simulink model "fitts_bimanual"  (Simulink 7.0)
settings: Solver=ode4  SolverMode=SingleTasking  StartTime=0.0  StopTime=inf  FixedStep=0.0005  RelTol=1e-3
undefined symbols (not defined in the file or in its folder): slselsubs
libraries: dspbuff3 x2, General x2, Video x1
settings Model: Creator=Administrator  LastModifiedBy=Administrator  BufferReuse=off
settings OptimizationCC: BlockReduction=off  OptimizeBlockIOStorage=off  BufferReuse=off  ExpressionFolding=off  LocalBlockOutputs=off
settings HardwareCC: ProdIntDivRoundTo=Floor  ProdEndianess=LittleEndian  ProdHWDeviceType=Intel->x86/Pentium  TargetHWDeviceType=32-bit Generic  ProdEqTarget=off
settings RTWCC: SystemTargetFile=xpctarget.tlc  TemplateMakefile=xpc_default_tmf  Description=xPC Target  ProcessScript=xpctarget_make_rtw_hook
settings xpcTargetCC: TargetFcnLib=ansi_tfl_table_tmw.mat  GenFloatMathFcnCalls=ANSI_C  CompOptLevelCompliant=off  PortableWordSizes=off  xPCisDownloadable=off

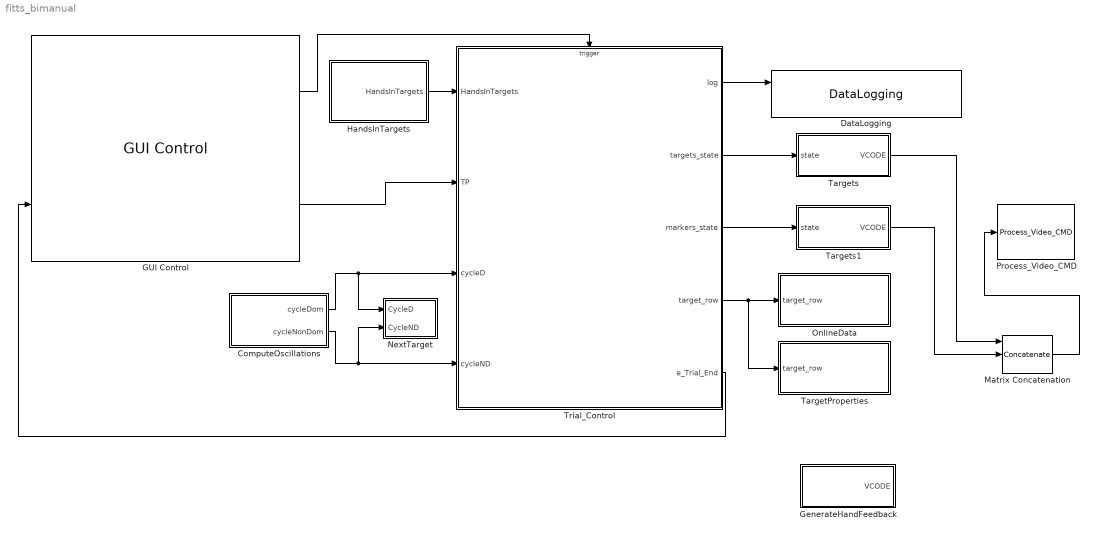
== system fitts_bimanual ==
  ComputeOscillations : Subsystem
  DataLogging : General/DataLogging  SystemSampleTime=-1  log_event_codes=on  log_analog_inputs=off
  GUI Control : General/GUI Control  SystemSampleTime=-1  target_type_str=Circle  Target_Type=1  XYcols=[1 2]  Vcols=3  Lcols=4  indices_padding=[0 0 0 0;0 0 0 0]  show_repeat_trial_flag=on
  GenerateHandFeedback : Subsystem
  HandsInTargets : Subsystem
  Matrix Concatenation : Concatenate  NumInputs=3  Mode=Multidimensional array
  NextTarget : Subsystem
  OnlineData : Subsystem
  Process_Video_CMD : Video/Process_Video_CMD  SystemSampleTime=-1
  TargetProperties : Subsystem
  Targets : Subsystem
  Targets1 : Subsystem
  Trial_Control : Stateflow chart
  wires:
  Matrix Concatenation/1 -> Process_Video_CMD/1
  Targets/1(VCODE) -> Matrix Concatenation/1
  GUI Control/1 -> Trial_Control/Trigger
  Trial_Control/5(e_Trial_End) -> GUI Control/2
  HandsInTargets/1(HandsInTargets) -> Trial_Control/1(HandsInTargets)
  GUI Control/2 -> Trial_Control/2(TP)
  Targets1/1(VCODE) -> Matrix Concatenation/2
  Trial_Control/2(targets_state) -> Targets/1(state)
  Trial_Control/3(markers_state) -> Targets1/1(state)
  Trial_Control/1(log) -> DataLogging/1
  ComputeOscillations/2(cycleNonDom) -> Trial_Control/4(cycleND), NextTarget/2(CycleND)
  ComputeOscillations/1(cycleDom) -> Trial_Control/3(cycleD), NextTarget/1(CycleD)
  Trial_Control/4(target_row) -> TargetProperties/1(target_row), OnlineData/1(target_row)

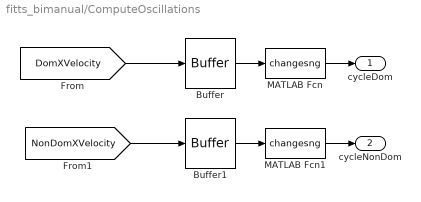
== system fitts_bimanual/ComputeOscillations ==
  Buffer : dspbuff3/Buffer  N=10  V=10  ic=0
  Buffer1 : dspbuff3/Buffer  N=10  V=10  ic=0
  MATLAB Fcn : MATLABFcn  MATLABFcn=changesng
  MATLAB Fcn1 : MATLABFcn  MATLABFcn=changesng
  cycleDom : Outport  OutDataType=sfix(16)  OutScaling=2^0
  cycleNonDom : Outport  Port=2  OutDataType=sfix(16)  OutScaling=2^0
  wires:
  Buffer/1 -> MATLAB Fcn/1
  MATLAB Fcn/1 -> cycleDom/1
  Buffer1/1 -> MATLAB Fcn1/1
  MATLAB Fcn1/1 -> cycleNonDom/1
  [DomXVelocity] -> Buffer/1
  [NonDomXVelocity] -> Buffer1/1

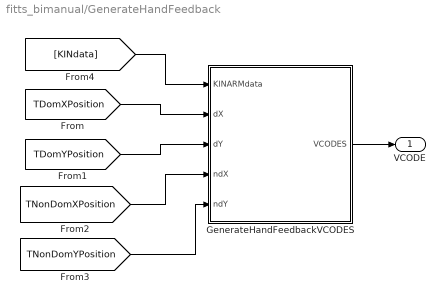
== system fitts_bimanual/GenerateHandFeedback ==
  GenerateHandFeedbackVCODES : Stateflow chart
  VCODE : Outport
  wires:
  GenerateHandFeedbackVCODES/1(VCODES) -> VCODE/1
  [KINdata] -> GenerateHandFeedbackVCODES/1(KINARMdata)
  [TDomXPosition] -> GenerateHandFeedbackVCODES/2(dX)
  [TDomYPosition] -> GenerateHandFeedbackVCODES/3(dY)
  [TNonDomXPosition] -> GenerateHandFeedbackVCODES/4(ndX)
  [TNonDomYPosition] -> GenerateHandFeedbackVCODES/5(ndY)

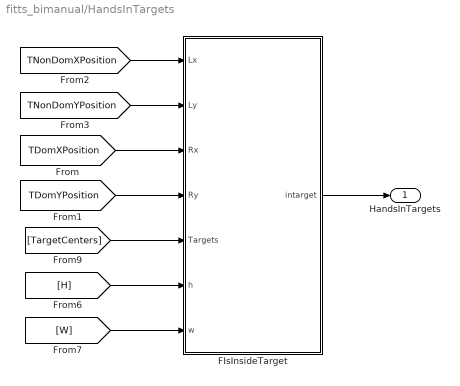
== system fitts_bimanual/HandsInTargets ==
  FIsInsideTarget : Stateflow chart
  HandsInTargets : Outport
  wires:
  [TargetCenters] -> FIsInsideTarget/5(Targets)
  [H] -> FIsInsideTarget/6(h)
  [W] -> FIsInsideTarget/7(w)
  FIsInsideTarget/1(intarget) -> HandsInTargets/1
  [TNonDomXPosition] -> FIsInsideTarget/1(Lx)
  [TNonDomYPosition] -> FIsInsideTarget/2(Ly)
  [TDomXPosition] -> FIsInsideTarget/3(Rx)
  [TDomYPosition] -> FIsInsideTarget/4(Ry)

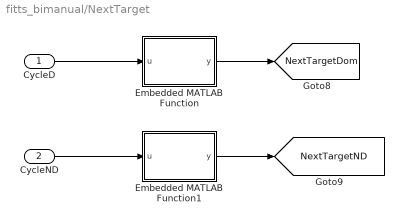
== system fitts_bimanual/NextTarget ==
  CycleD : Inport
  CycleND : Inport  Port=2
  Embedded MATLAB Function : Stateflow chart
  Embedded MATLAB Function1 : Stateflow chart
  tag scope: NextTargetDom=global, NextTargetND=global
  wires:
  CycleD/1 -> Embedded MATLAB Function/1(u)
  CycleND/1 -> Embedded MATLAB Function1/1(u)
  Embedded MATLAB Function/1(y) -> [NextTargetDom]
  Embedded MATLAB Function1/1(y) -> [NextTargetND]

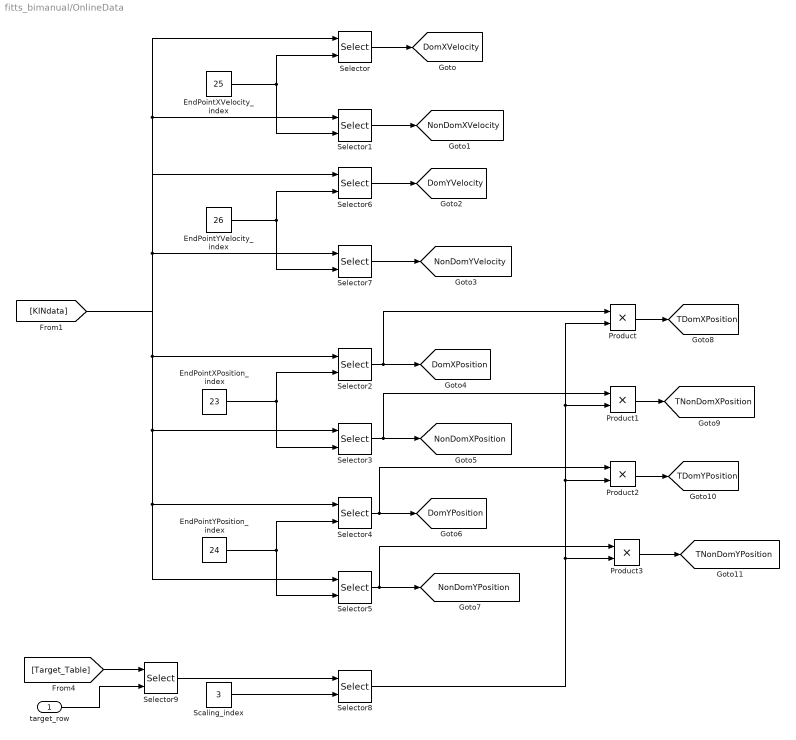
== system fitts_bimanual/OnlineData ==
  target_row : Inport  OutDataType=sfix(16)  OutScaling=2^0
  EndPointXPosition_index : Constant  Value=23  OutDataType=sfix(16)  OutScaling=2^0
  EndPointXVelocity_index : Constant  Value=25  OutDataType=sfix(16)  OutScaling=2^0
  EndPointYPosition_index : Constant  Value=24  OutDataType=sfix(16)  OutScaling=2^0
  EndPointYVelocity_index : Constant  Value=26  OutDataType=sfix(16)  OutScaling=2^0
  Product{,1..3} (4 alike) : Product  OutDataType=sfix(16)  OutScaling=2^0  RndMeth=Zero
  Scaling_index : Constant  Value=3  OutDataType=sfix(16)  OutScaling=2^0
  Selector{,2,4,6,8..9} (6 alike) : Selector  NumberOfDimensions=2  InputPortWidth=3  IndexOptions=Index vector (port),Index vector (dialog)  Indices=1,1  OutputSizes=slselsubs([(-2),(-2)],1),slselsubs([(-2),(-2)],2)
  Selector{1,3,5,7} (4 alike) : Selector  NumberOfDimensions=2  InputPortWidth=3  IndexOptions=Index vector (port),Index vector (dialog)  Indices=1,2  OutputSizes=slselsubs([(-2),(-2)],1),slselsubs([(-2),(-2)],2)
  tag scope: DomXPosition=global, DomXVelocity=global, DomYPosition=global, DomYVelocity=global, NonDomXPosition=global, NonDomXVelocity=global, NonDomYPosition=global, NonDomYVelocity=global, TDomXPosition=global, TDomYPosition=global, TNonDomXPosition=global, TNonDomYPosition=global
  wires:
  [KINdata] -> Selector1/1, Selector/1, Selector2/1, Selector3/1, Selector4/1, Selector5/1, Selector6/1, Selector7/1
  Selector3/1 -> [NonDomXPosition], Product1/1
  Selector/1 -> [DomXVelocity]
  EndPointXVelocity_index/1 -> Selector/2, Selector1/2
  Selector1/1 -> [NonDomXVelocity]
  EndPointXPosition_index/1 -> Selector2/2, Selector3/2
  Selector2/1 -> [DomXPosition], Product/1
  Selector5/1 -> [NonDomYPosition], Product3/1
  EndPointYPosition_index/1 -> Selector4/2, Selector5/2
  Selector4/1 -> [DomYPosition], Product2/1
  Selector6/1 -> [DomYVelocity]
  EndPointYVelocity_index/1 -> Selector6/2, Selector7/2
  Selector7/1 -> [NonDomYVelocity]
  Product/1 -> [TDomXPosition]
  Product1/1 -> [TNonDomXPosition]
  Product2/1 -> [TDomYPosition]
  Product3/1 -> [TNonDomYPosition]
  Scaling_index/1 -> Selector8/2
  Selector8/1 -> Product/2, Product1/2, Product2/2, Product3/2
  Selector9/1 -> Selector8/1
  [Target_Table] -> Selector9/1
  target_row/1 -> Selector9/2

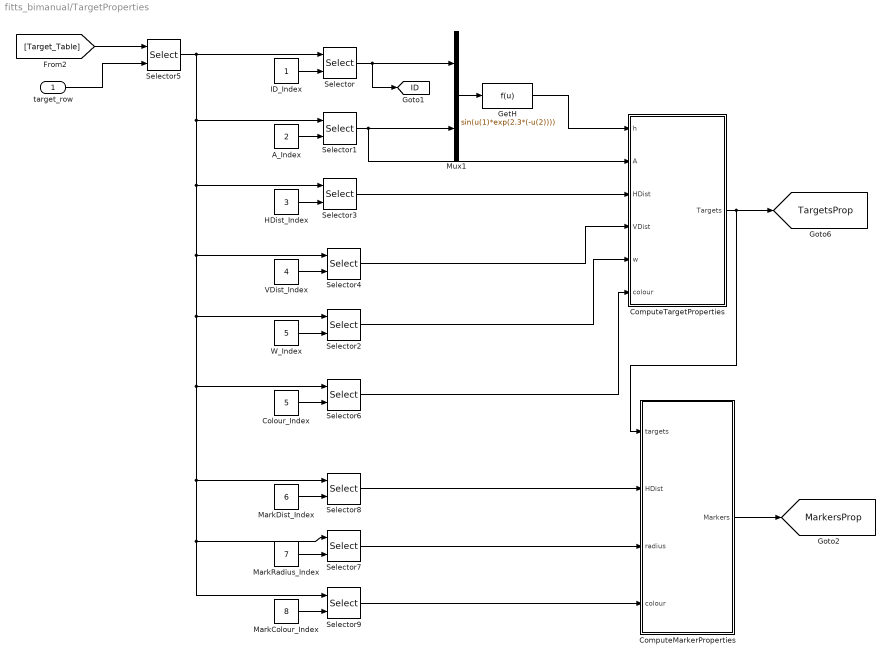
== system fitts_bimanual/TargetProperties ==
  target_row : Inport  OutDataType=sfix(16)  OutScaling=2^0
  A_Index : Constant  Value=2  OutDataType=sfix(16)  OutScaling=2^0
  Colour_Index : Constant  Value=5  OutDataType=sfix(16)  OutScaling=2^0
  ComputeMarkerProperties : Stateflow chart
  ComputeTargetProperties : Stateflow chart
  GetH : Fcn  Expr=sin(u(1)*exp(2.3*(-u(2))))
  HDist_Index : Constant  Value=3  OutDataType=sfix(16)  OutScaling=2^0
  ID_Index : Constant  OutDataType=sfix(16)  OutScaling=2^0
  MarkColour_Index : Constant  Value=8  OutDataType=sfix(16)  OutScaling=2^0
  MarkDist_Index : Constant  Value=6  OutDataType=sfix(16)  OutScaling=2^0
  MarkRadius_Index : Constant  Value=7  OutDataType=sfix(16)  OutScaling=2^0
  Mux1 : Mux  Inputs=2
  Selector{,1..9} (10 alike) : Selector  NumberOfDimensions=2  InputPortWidth=3  IndexOptions=Index vector (port),Index vector (dialog)  Indices=1,1  OutputSizes=slselsubs([(-2),(-2)],1),slselsubs([(-2),(-2)],2)
  VDist_Index : Constant  Value=4  OutDataType=sfix(16)  OutScaling=2^0
  W_Index : Constant  Value=5  OutDataType=sfix(16)  OutScaling=2^0
  tag scope: ID=global, MarkersProp=global, TargetsProp=global
  wires:
  ID_Index/1 -> Selector/2
  Selector5/1 -> Selector/1, Selector1/1, Selector3/1, Selector4/1, Selector2/1, Selector6/1, Selector8/1, Selector7/1, Selector9/1
  A_Index/1 -> Selector1/2
  HDist_Index/1 -> Selector3/2
  VDist_Index/1 -> Selector4/2
  Mux1/1 -> GetH/1
  Selector/1 -> Mux1/1, [ID]
  Selector1/1 -> Mux1/2, ComputeTargetProperties/2(A)
  Selector3/1 -> ComputeTargetProperties/3(HDist)
  Selector4/1 -> ComputeTargetProperties/4(VDist)
  ComputeTargetProperties/1(Targets) -> [TargetsProp], ComputeMarkerProperties/1(targets)
  W_Index/1 -> Selector2/2
  Selector2/1 -> ComputeTargetProperties/5(w)
  Colour_Index/1 -> Selector6/2
  Selector6/1 -> ComputeTargetProperties/6(colour)
  GetH/1 -> ComputeTargetProperties/1(h)
  [Target_Table] -> Selector5/1
  target_row/1 -> Selector5/2
  MarkDist_Index/1 -> Selector8/2
  MarkRadius_Index/1 -> Selector7/2
  MarkColour_Index/1 -> Selector9/2
  Selector8/1 -> ComputeMarkerProperties/2(HDist)
  Selector7/1 -> ComputeMarkerProperties/3(radius)
  Selector9/1 -> ComputeMarkerProperties/4(colour)
  ComputeMarkerProperties/1(Markers) -> [MarkersProp]

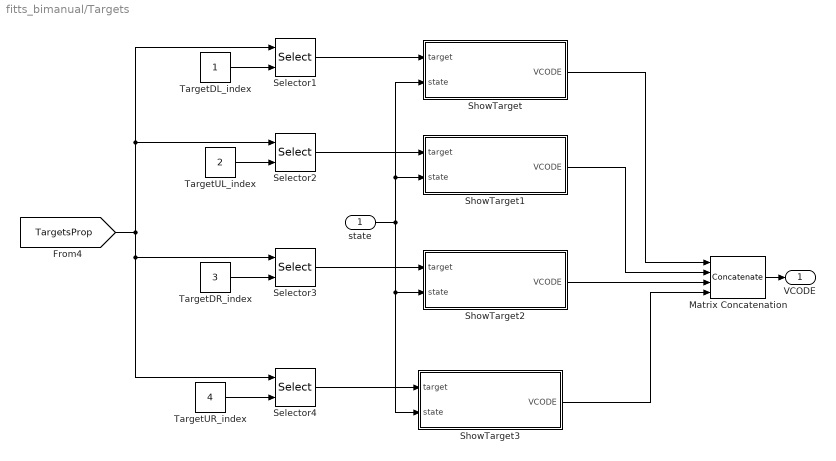
== system fitts_bimanual/Targets ==
  state : Inport
  Matrix Concatenation : Concatenate  NumInputs=4  Mode=Multidimensional array
  Selector{1..4} (4 alike) : Selector  NumberOfDimensions=2  InputPortWidth=3  IndexOptions=Index vector (port),Index vector (dialog)  Indices=1,2  OutputSizes=slselsubs([(-2),(-2)],1),slselsubs([(-2),(-2)],2)
  ShowTarget : Stateflow chart
  ShowTarget1 : Stateflow chart
  ShowTarget2 : Stateflow chart
  ShowTarget3 : Stateflow chart
  TargetDL_index : Constant  OutDataType=sfix(16)  OutScaling=2^0
  TargetDR_index : Constant  Value=3  OutDataType=sfix(16)  OutScaling=2^0
  TargetUL_index : Constant  Value=2  OutDataType=sfix(16)  OutScaling=2^0
  TargetUR_index : Constant  Value=4  OutDataType=sfix(16)  OutScaling=2^0
  VCODE : Outport  OutDataType=sfix(16)  OutScaling=2^0
  wires:
  state/1 -> ShowTarget/2(state), ShowTarget1/2(state), ShowTarget2/2(state), ShowTarget3/2(state)
  ShowTarget/1(VCODE) -> Matrix Concatenation/1
  ShowTarget1/1(VCODE) -> Matrix Concatenation/2
  ShowTarget2/1(VCODE) -> Matrix Concatenation/3
  Matrix Concatenation/1 -> VCODE/1
  ShowTarget3/1(VCODE) -> Matrix Concatenation/4
  TargetDL_index/1 -> Selector1/2
  [TargetsProp] -> Selector1/1, Selector2/1, Selector3/1, Selector4/1
  TargetUL_index/1 -> Selector2/2
  TargetDR_index/1 -> Selector3/2
  TargetUR_index/1 -> Selector4/2
  Selector1/1 -> ShowTarget/1(target)
  Selector2/1 -> ShowTarget1/1(target)
  Selector3/1 -> ShowTarget2/1(target)
  Selector4/1 -> ShowTarget3/1(target)

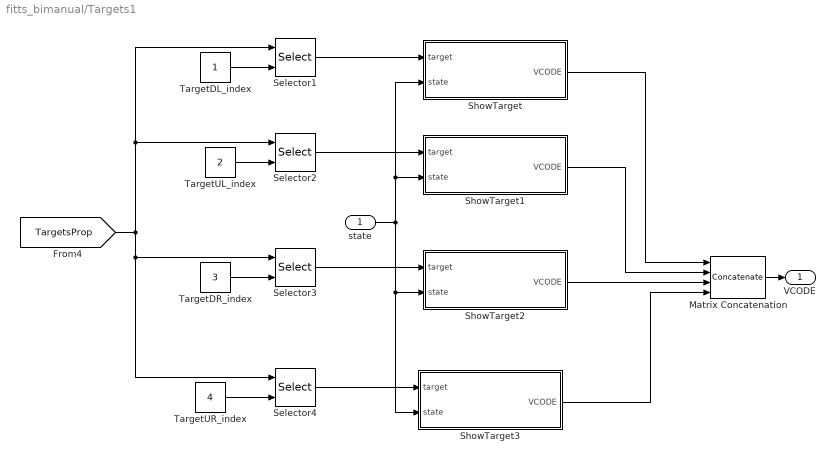
== system fitts_bimanual/Targets1 ==
  state : Inport
  Matrix Concatenation : Concatenate  NumInputs=4  Mode=Multidimensional array
  Selector{1..4} (4 alike) : Selector  NumberOfDimensions=2  InputPortWidth=3  IndexOptions=Index vector (port),Index vector (dialog)  Indices=1,2  OutputSizes=slselsubs([(-2),(-2)],1),slselsubs([(-2),(-2)],2)
  ShowTarget : Stateflow chart
  ShowTarget1 : Stateflow chart
  ShowTarget2 : Stateflow chart
  ShowTarget3 : Stateflow chart
  TargetDL_index : Constant  OutDataType=sfix(16)  OutScaling=2^0
  TargetDR_index : Constant  Value=3  OutDataType=sfix(16)  OutScaling=2^0
  TargetUL_index : Constant  Value=2  OutDataType=sfix(16)  OutScaling=2^0
  TargetUR_index : Constant  Value=4  OutDataType=sfix(16)  OutScaling=2^0
  VCODE : Outport  OutDataType=sfix(16)  OutScaling=2^0
  wires:
  state/1 -> ShowTarget/2(state), ShowTarget1/2(state), ShowTarget2/2(state), ShowTarget3/2(state)
  ShowTarget/1(VCODE) -> Matrix Concatenation/1
  ShowTarget1/1(VCODE) -> Matrix Concatenation/2
  ShowTarget2/1(VCODE) -> Matrix Concatenation/3
  Matrix Concatenation/1 -> VCODE/1
  ShowTarget3/1(VCODE) -> Matrix Concatenation/4
  TargetDL_index/1 -> Selector1/2
  [TargetsProp] -> Selector1/1, Selector2/1, Selector3/1, Selector4/1
  TargetUL_index/1 -> Selector2/2
  TargetDR_index/1 -> Selector3/2
  TargetUR_index/1 -> Selector4/2
  Selector1/1 -> ShowTarget/1(target)
  Selector2/1 -> ShowTarget1/1(target)
  Selector3/1 -> ShowTarget2/1(target)
  Selector4/1 -> ShowTarget3/1(target)

== stateflow chart Trial_Control ==
  state Initialize/
    log=0
  state Wait4Subject/
    //Turn on markers and targets with specified size
    targets_state=1
    markers_state=1
    log=0
    oscillations=0
  state PreOscillationDelay/
    //Wait specified period of time
    delay=TP[0]
  state Oscillate/
    //Hold oscillation until subject reaches trial limit
    markers_state=0
    log=1
  state EndOfTrial/
    //Wait specified period of time
    delay=TP[0]
    targets_state=0
  state InterTrial/
    //Set up new
    e_Trial_End
    delay=TP[0]
  Wait4Subject -> PreOscillationDelay : [HandsInTargets]
  PreOscillationDelay -> Oscillate : after(delay,e_clk)
  Initialize -> Wait4Subject
  Oscillate -> EndOfTrial : [oscillations=TP[0]]
  EndOfTrial -> InterTrial
  InterTrial -> Wait4Subject : after(delay,e_clk)
  (default) -> Initialize : //init task
  data: log output boolean; HandsInTargets input inherited; TP input inherited; cycleD input inherited; targets_state output boolean; markers_state output double; cycleND input inherited; PREOSCDELAY_COL constant uint8 =1; INTERTRIALDELAY_COL constant uint8 =2; FEEDBACKSCALING_COL constant uint8 =3; target_row output double
  events: e_clk input RISING_EDGE_EVENT; e_ExitTrialNow input EITHER_EDGE_EVENT; e_Trial_End output EITHER_EDGE_EVENT

== matlab function NextTarget/Embedded MATLAB Function ==
  data: u input inherited; y output inherited
function y = fcn(u)
% This block supports the Embedded MATLAB subset.
% See the help menu for details. 

y = u;

== matlab function NextTarget/Embedded MATLAB Function1 ==
  data: u input inherited; y output inherited
function y = fcn(u)
% This block supports the Embedded MATLAB subset.
% See the help menu for details. 

y = u;

== matlab function GenerateHandFeedback/GenerateHandFeedbackVCODES ==
  data: KINARMdata input inherited; VCODES output inherited; dX input inherited; dY input inherited; ndX input inherited; ndY input inherited
function VCODES  = fcn(KINARMdata,dX,dY,ndX,ndY)
%
% This function creates the VCODEs for the hand position feedback for both
% hands.  Various options in the Mask of the Simulink block in which this
% embedded Matlab file sits, allow the user to specify how often
% the hand feedback is updated as well as the source of the style and status
% of the hand feedback.  


dominant_arm=KINARMdata(3,1);
feedfwd=KINARMdata(3,2);				%amount of feedforward extrapolation for hand position(s)
fdbk_stts_GUI=KINARMdata(3,3);			%status of hand feedback requested from GUI
fdbk_src_GUI=KINARMdata(3,4);			%source of hand feedback style requested from GUI
fdbk_clr_GUI=KINARMdata(3,5);			%colour of hand feedback required by GUI
fdbk_radius_GUI=KINARMdata(3,6);		%radius of hand feedback required by GUI


%----------------Feedback Style ----------------
VCODES=zeros(2,20);						%set default
VCODES(:,1)=1;							%target_type of circle
VCODES(:,5)=fdbk_clr_GUI;				%fill colour as specified by GUI
VCODES(:,6)=fdbk_clr_GUI;				%stroke colour same as fill colour
VCODES(:,7)=0;							%no stroke width
VCODES(:,10)=fdbk_radius_GUI;			%radius (m) as specified by GUI

%show both hand feedbacks
VCODES(1,2)=1;
VCODES(2,2)=1;
end

%----------------Feedback Position ----------------
%set the position of the hand feedback.
for i=1:2
	if i==1
		active_arm=KINARMdata(3,1);			%choose dominant arm first
	else
		active_arm=3-KINARMdata(3,1);		%choose non-dominant arm 2nd
	end
	HandXPos=KINARMdata(active_arm,23);		%(m)
	HandYPos=KINARMdata(active_arm,24);		%(m)
	HandXVel=KINARMdata(active_arm,25);		%(m/s)
	HandYVel=KINARMdata(active_arm,26);		%(m/s)

	% feed-forward hand position (m)
	HandXPos_ff = HandXPos + HandXVel*feedfwd;
	HandYPos_ff = HandYPos + HandYVel*feedfwd;
	VCODES(i,3)=HandXPos_ff;				%target position in m 
	VCODES(i,4)=HandYPos_ff;				%target position in m 
end

VCODES_out=VCODES;

== matlab function TargetProperties/ComputeMarkerProperties ==
  data: targets input inherited; HDist input inherited; radius input inherited; Markers output inherited; colour input inherited
function Markers = fcn(targets,HDist,radius,colour)
% This block supports the Embedded MATLAB subset.
% See the help menu for details. 

% Components of the returned arrays: FORGET ABOUT IT!!!
% X0[1,:] -> Dominant arm
% X0[2,:] -> Non Dominant arm
% X0[:,1] -> Lower targets
% X0[:,2] -> Upper targets

% New version:
% Targets:[ x1, y1, w, h, colour]  Left Down
%         [ x2, y2, w, h, colour]  Left Up
%         [ x3, y3, w, h, colour]  Right Down
%         [ x4, y4, w, h, colour]  Right Up

c=1;  % Distances are in centimeters, need to convert to meters. CHECK UNITS!!!!!

Targets = [ -HDist/2*c, VDist*c,     w, h, colour; ...
            -HDist/2*c, VDist*c+A*c, w, h, colour; ...
             HDist/2*c, VDist*c,     w, h, colour; ...
             HDist/2*c, VDist*c+A*c, w, h, colour];

== matlab function HandsInTargets/FIsInsideTarget ==
  data: Lx input inherited; Ly input inherited; Rx input inherited; Ry input inherited; Targets input inherited; h input inherited; intarget output inherited; w input inherited
function intarget = fcn(Lx,Ly,Rx,Ry,Targets,h,w)
% This block supports the Embedded MATLAB subset.
% See the help menu for details. 

 deltaLx = Lx - Targets(:,1)*0.01;
 deltaLy = Ly - Targets(:,2)*0.01;
 deltaRx = Rx - Targets(:,1)*0.01;
 deltaRy = Ry - Targets(:,2)*0.01;
 
 intarget = zeros(length(Targets),2);
 
 intarget(:,1)= abs(deltaLx) <= w/2 & abs(deltaLy) <= h/2;
 intarget(:,2)= abs(deltaRx) <= w/2 & abs(deltaRy) <= h/2;

== matlab function Targets/ShowTarget1 ==
  data: target input inherited; VCODE output inherited; state input inherited
function VCODE  = fcn(target, state)
% This block supports an embeddable subset of the MATLAB language.
% See the help menu for details. 

% VCODEs are length 20.
% All dimensions are units of (m).
% VCODE index definition: 1-5 as the same for all target types
% 1 - Target type
%		1=circle
%		2=ellipse
%       3=rectangle
%		4=line
%       5=triangle
%		6 and higher - not implemented yet
% 2 - status
%		0=off
%		1=on
% 3 - x position (m)
% 4 - y position (m)
% 5 - fill colour
% 6 - stroke colour
% 7 - stroke width
% 8 - reserved
% 9 - reserved
%
% For circles
% 10 - radius (m)
%
% For ellipses
% 10 - major radius (m)
% 11 - minor radius (m)
% 12 - orientation of major axis (rad)
%
% For rectangles
% 10 - length (m)
% 11 - height (m)
% 12 - orientation (rad) (relative to x,y already shown)
%
% For lines
% 10 - end point x-axis coordinate relative to start point (m)
% 11 - end point y-axis coordinate relative to start point (m)
%
% For triangles
% 10 - length (m)
% 11 - height (m)
% 12 - offset of peak from midpoint of length (m)
% 13 - orientation (rad)

VCODE=zeros(1,20);		%default - target is not defined

if (state==0)
	return;							%state==0 means that the target is off
end

VCODE(1)=3; %They are rectangles

VCODE(2)=1;							%default is that target is 'on'
VCODE(3)=target_pos(0)*0.01;		%target position in target table is cm (v1.4)
VCODE(4)=target_pos(1)*0.01;		%target position in target table is cm (v1.4)

% Fill colour currently comes from the GUI in 1.x format: RRRGGGBBB. Convert this to a 32-bit 
% 0xRRGGBBAA value, or use zero for transparency if target table index for the colour is zero.
if stateindices(state,1)==0
	VCODE(5)=0;
else
	VCODE(5)=colourshift(target(5));			%fill colour
end

% Stroke colour currently comes from the GUI in 1.x format: RRRGGGBBB. Convert this to a 32-bit 
% 0xRRGGBBAA value, or use zero for transparency if target table index for the colour is zero.
% if stateindices(state,2)==0
% 	VCODE(6)=0;				%if stroke-colour column==0, then stroke colour=0
% else
% 	VCODE(6)=colourshift(target(stateindices(state,2)));			%stroke colour
% end

%if target table index for stroke width is zero, then the stroke width is undefined
% if stateindices(state,3)==0
% 	VCODE(7)=0;					%if stroke-width column==0, then stroke width=0
% elseif stateindices(state,3)<0
% 	VCODE(7)=0.001;			%if stroke is not defined, then a 1mm default is chosen
% else
% 	VCODE(7)=target(stateindices(state,3))*0.01;	%stroke width in target table is cm 
% end

VCODE(10)=target(3)*0.01;       %length (m) -- length in target table is in cm
VCODE(11)=target(4)*0.01;       %height (m) -- height in target table is in cm
% if stateindices(state,6)==0
%     VCODE(12)=0;				%if orientation column==0, then orientation=0
% else
%     VCODE(12)=mod(target(stateindices(state,6)),360)*pi/180.0;  %orientation (rad) -- orientation in target table is degrees (v1.4)
% end

%colourshift converts an RRRGGGBBB colour into an RRGBBAA, as an uint32 
function RRGGBBAA = colourshift(RRRGGGBBB)
	blue = cast(mod(RRRGGGBBB,1000),'uint32');
	green= cast(mod(RRRGGGBBB-blue,1000000)/1000,'uint32');
	red  = cast((RRRGGGBBB-green*1000-blue)/1000000,'uint32');
    RRGGBBAA =   bitshift(red,24)...		% red component
				+ bitshift(green,16)...		% green component
				+ bitshift(blue,8)...		% blue component
				+ 255;						% alpha component

== matlab function Targets/ShowTarget2 ==
  data: target input inherited; VCODE output inherited; state input inherited
function VCODE  = fcn(target, state)
% This block supports an embeddable subset of the MATLAB language.
% See the help menu for details. 

% VCODEs are length 20.
% All dimensions are units of (m).
% VCODE index definition: 1-5 as the same for all target types
% 1 - Target type
%		1=circle
%		2=ellipse
%       3=rectangle
%		4=line
%       5=triangle
%		6 and higher - not implemented yet
% 2 - status
%		0=off
%		1=on
% 3 - x position (m)
% 4 - y position (m)
% 5 - fill colour
% 6 - stroke colour
% 7 - stroke width
% 8 - reserved
% 9 - reserved
%
% For circles
% 10 - radius (m)
%
% For ellipses
% 10 - major radius (m)
% 11 - minor radius (m)
% 12 - orientation of major axis (rad)
%
% For rectangles
% 10 - length (m)
% 11 - height (m)
% 12 - orientation (rad) (relative to x,y already shown)
%
% For lines
% 10 - end point x-axis coordinate relative to start point (m)
% 11 - end point y-axis coordinate relative to start point (m)
%
% For triangles
% 10 - length (m)
% 11 - height (m)
% 12 - offset of peak from midpoint of length (m)
% 13 - orientation (rad)

VCODE=zeros(1,20);		%default - target is not defined

if (state==0)
	return;							%state==0 means that the target is off
end

VCODE(1)=3; %They are rectangles

VCODE(2)=1;							%default is that target is 'on'
VCODE(3)=target_pos(0)*0.01;		%target position in target table is cm (v1.4)
VCODE(4)=target_pos(1)*0.01;		%target position in target table is cm (v1.4)

% Fill colour currently comes from the GUI in 1.x format: RRRGGGBBB. Convert this to a 32-bit 
% 0xRRGGBBAA value, or use zero for transparency if target table index for the colour is zero.
if stateindices(state,1)==0
	VCODE(5)=0;
else
	VCODE(5)=colourshift(target(5));			%fill colour
end

% Stroke colour currently comes from the GUI in 1.x format: RRRGGGBBB. Convert this to a 32-bit 
% 0xRRGGBBAA value, or use zero for transparency if target table index for the colour is zero.
% if stateindices(state,2)==0
% 	VCODE(6)=0;				%if stroke-colour column==0, then stroke colour=0
% else
% 	VCODE(6)=colourshift(target(stateindices(state,2)));			%stroke colour
% end

%if target table index for stroke width is zero, then the stroke width is undefined
% if stateindices(state,3)==0
% 	VCODE(7)=0;					%if stroke-width column==0, then stroke width=0
% elseif stateindices(state,3)<0
% 	VCODE(7)=0.001;			%if stroke is not defined, then a 1mm default is chosen
% else
% 	VCODE(7)=target(stateindices(state,3))*0.01;	%stroke width in target table is cm 
% end

VCODE(10)=target(3)*0.01;       %length (m) -- length in target table is in cm
VCODE(11)=target(4)*0.01;       %height (m) -- height in target table is in cm
% if stateindices(state,6)==0
%     VCODE(12)=0;				%if orientation column==0, then orientation=0
% else
%     VCODE(12)=mod(target(stateindices(state,6)),360)*pi/180.0;  %orientation (rad) -- orientation in target table is degrees (v1.4)
% end

%colourshift converts an RRRGGGBBB colour into an RRGBBAA, as an uint32 
function RRGGBBAA = colourshift(RRRGGGBBB)
	blue = cast(mod(RRRGGGBBB,1000),'uint32');
	green= cast(mod(RRRGGGBBB-blue,1000000)/1000,'uint32');
	red  = cast((RRRGGGBBB-green*1000-blue)/1000000,'uint32');
    RRGGBBAA =   bitshift(red,24)...		% red component
				+ bitshift(green,16)...		% green component
				+ bitshift(blue,8)...		% blue component
				+ 255;						% alpha component

== matlab function Targets/ShowTarget3 ==
  data: target input inherited; VCODE output inherited; state input inherited
function VCODE  = fcn(target, state)
% This block supports an embeddable subset of the MATLAB language.
% See the help menu for details. 

% VCODEs are length 20.
% All dimensions are units of (m).
% VCODE index definition: 1-5 as the same for all target types
% 1 - Target type
%		1=circle
%		2=ellipse
%       3=rectangle
%		4=line
%       5=triangle
%		6 and higher - not implemented yet
% 2 - status
%		0=off
%		1=on
% 3 - x position (m)
% 4 - y position (m)
% 5 - fill colour
% 6 - stroke colour
% 7 - stroke width
% 8 - reserved
% 9 - reserved
%
% For circles
% 10 - radius (m)
%
% For ellipses
% 10 - major radius (m)
% 11 - minor radius (m)
% 12 - orientation of major axis (rad)
%
% For rectangles
% 10 - length (m)
% 11 - height (m)
% 12 - orientation (rad) (relative to x,y already shown)
%
% For lines
% 10 - end point x-axis coordinate relative to start point (m)
% 11 - end point y-axis coordinate relative to start point (m)
%
% For triangles
% 10 - length (m)
% 11 - height (m)
% 12 - offset of peak from midpoint of length (m)
% 13 - orientation (rad)

VCODE=zeros(1,20);		%default - target is not defined

if (state==0)
	return;							%state==0 means that the target is off
end

VCODE(1)=3; %They are rectangles

VCODE(2)=1;							%default is that target is 'on'
VCODE(3)=target_pos(0)*0.01;		%target position in target table is cm (v1.4)
VCODE(4)=target_pos(1)*0.01;		%target position in target table is cm (v1.4)

% Fill colour currently comes from the GUI in 1.x format: RRRGGGBBB. Convert this to a 32-bit 
% 0xRRGGBBAA value, or use zero for transparency if target table index for the colour is zero.
if stateindices(state,1)==0
	VCODE(5)=0;
else
	VCODE(5)=colourshift(target(5));			%fill colour
end

% Stroke colour currently comes from the GUI in 1.x format: RRRGGGBBB. Convert this to a 32-bit 
% 0xRRGGBBAA value, or use zero for transparency if target table index for the colour is zero.
% if stateindices(state,2)==0
% 	VCODE(6)=0;				%if stroke-colour column==0, then stroke colour=0
% else
% 	VCODE(6)=colourshift(target(stateindices(state,2)));			%stroke colour
% end

%if target table index for stroke width is zero, then the stroke width is undefined
% if stateindices(state,3)==0
% 	VCODE(7)=0;					%if stroke-width column==0, then stroke width=0
% elseif stateindices(state,3)<0
% 	VCODE(7)=0.001;			%if stroke is not defined, then a 1mm default is chosen
% else
% 	VCODE(7)=target(stateindices(state,3))*0.01;	%stroke width in target table is cm 
% end

VCODE(10)=target(3)*0.01;       %length (m) -- length in target table is in cm
VCODE(11)=target(4)*0.01;       %height (m) -- height in target table is in cm
% if stateindices(state,6)==0
%     VCODE(12)=0;				%if orientation column==0, then orientation=0
% else
%     VCODE(12)=mod(target(stateindices(state,6)),360)*pi/180.0;  %orientation (rad) -- orientation in target table is degrees (v1.4)
% end

%colourshift converts an RRRGGGBBB colour into an RRGBBAA, as an uint32 
function RRGGBBAA = colourshift(RRRGGGBBB)
	blue = cast(mod(RRRGGGBBB,1000),'uint32');
	green= cast(mod(RRRGGGBBB-blue,1000000)/1000,'uint32');
	red  = cast((RRRGGGBBB-green*1000-blue)/1000000,'uint32');
    RRGGBBAA =   bitshift(red,24)...		% red component
				+ bitshift(green,16)...		% green component
				+ bitshift(blue,8)...		% blue component
				+ 255;						% alpha component

== matlab function Targets/ShowTarget ==
  data: target input inherited; VCODE output inherited; state input inherited
function VCODE  = fcn(target, state)
% This block supports an embeddable subset of the MATLAB language.
% See the help menu for details. 

% VCODEs are length 20.
% All dimensions are units of (m).
% VCODE index definition: 1-5 as the same for all target types
% 1 - Target type
%		1=circle
%		2=ellipse
%       3=rectangle
%		4=line
%       5=triangle
%		6 and higher - not implemented yet
% 2 - status
%		0=off
%		1=on
% 3 - x position (m)
% 4 - y position (m)
% 5 - fill colour
% 6 - stroke colour
% 7 - stroke width
% 8 - reserved
% 9 - reserved
%
% For circles
% 10 - radius (m)
%
% For ellipses
% 10 - major radius (m)
% 11 - minor radius (m)
% 12 - orientation of major axis (rad)
%
% For rectangles
% 10 - length (m)
% 11 - height (m)
% 12 - orientation (rad) (relative to x,y already shown)
%
% For lines
% 10 - end point x-axis coordinate relative to start point (m)
% 11 - end point y-axis coordinate relative to start point (m)
%
% For triangles
% 10 - length (m)
% 11 - height (m)
% 12 - offset of peak from midpoint of length (m)
% 13 - orientation (rad)

VCODE=zeros(1,20);		%default - target is not defined

if (state==0)
	return;							%state==0 means that the target is off
end

VCODE(1)=3; %They are rectangles

VCODE(2)=1;							%default is that target is 'on'
VCODE(3)=target_pos(0)*0.01;		%target position in target table is cm (v1.4)
VCODE(4)=target_pos(1)*0.01;		%target position in target table is cm (v1.4)

% Fill colour currently comes from the GUI in 1.x format: RRRGGGBBB. Convert this to a 32-bit 
% 0xRRGGBBAA value, or use zero for transparency if target table index for the colour is zero.
if stateindices(state,1)==0
	VCODE(5)=0;
else
	VCODE(5)=colourshift(target(5));			%fill colour
end

% Stroke colour currently comes from the GUI in 1.x format: RRRGGGBBB. Convert this to a 32-bit 
% 0xRRGGBBAA value, or use zero for transparency if target table index for the colour is zero.
% if stateindices(state,2)==0
% 	VCODE(6)=0;				%if stroke-colour column==0, then stroke colour=0
% else
% 	VCODE(6)=colourshift(target(stateindices(state,2)));			%stroke colour
% end

%if target table index for stroke width is zero, then the stroke width is undefined
% if stateindices(state,3)==0
% 	VCODE(7)=0;					%if stroke-width column==0, then stroke width=0
% elseif stateindices(state,3)<0
% 	VCODE(7)=0.001;			%if stroke is not defined, then a 1mm default is chosen
% else
% 	VCODE(7)=target(stateindices(state,3))*0.01;	%stroke width in target table is cm 
% end

VCODE(10)=target(3)*0.01;       %length (m) -- length in target table is in cm
VCODE(11)=target(4)*0.01;       %height (m) -- height in target table is in cm
% if stateindices(state,6)==0
%     VCODE(12)=0;				%if orientation column==0, then orientation=0
% else
%     VCODE(12)=mod(target(stateindices(state,6)),360)*pi/180.0;  %orientation (rad) -- orientation in target table is degrees (v1.4)
% end

%colourshift converts an RRRGGGBBB colour into an RRGBBAA, as an uint32 
function RRGGBBAA = colourshift(RRRGGGBBB)
	blue = cast(mod(RRRGGGBBB,1000),'uint32');
	green= cast(mod(RRRGGGBBB-blue,1000000)/1000,'uint32');
	red  = cast((RRRGGGBBB-green*1000-blue)/1000000,'uint32');
    RRGGBBAA =   bitshift(red,24)...		% red component
				+ bitshift(green,16)...		% green component
				+ bitshift(blue,8)...		% blue component
				+ 255;						% alpha component

== matlab function TargetProperties/ComputeTargetProperties ==
  data: h input inherited; A input inherited; Targets output inherited; HDist input inherited; VDist input inherited; w input inherited; colour input inherited
function Targets = fcn(h,A,HDist,VDist,w,colour)
% This block supports the Embedded MATLAB subset.
% See the help menu for details. 

% Components of the returned arrays: FORGET ABOUT IT!!!
% X0[1,:] -> Dominant arm
% X0[2,:] -> Non Dominant arm
% X0[:,1] -> Lower targets
% X0[:,2] -> Upper targets

% New version:
% Targets:[ x1, y1, w, h, colour]  Left Down
%         [ x2, y2, w, h, colour]  Left Up
%         [ x3, y3, w, h, colour]  Right Down
%         [ x4, y4, w, h, colour]  Right Up

c=1;  % Distances are in centimeters, need to convert to meters. CHECK UNITS!!!!!

Targets = [ -HDist/2*c, VDist*c,     w, h, colour; ...
            -HDist/2*c, VDist*c+A*c, w, h, colour; ...
             HDist/2*c, VDist*c,     w, h, colour; ...
             HDist/2*c, VDist*c+A*c, w, h, colour];

== matlab function Targets1/ShowTarget ==
  data: target input inherited; VCODE output inherited; state input inherited
function VCODE  = fcn(target, state)
% This block supports an embeddable subset of the MATLAB language.
% See the help menu for details. 

% VCODEs are length 20.
% All dimensions are units of (m).
% VCODE index definition: 1-5 as the same for all target types
% 1 - Target type
%		1=circle
%		2=ellipse
%       3=rectangle
%		4=line
%       5=triangle
%		6 and higher - not implemented yet
% 2 - status
%		0=off
%		1=on
% 3 - x position (m)
% 4 - y position (m)
% 5 - fill colour
% 6 - stroke colour
% 7 - stroke width
% 8 - reserved
% 9 - reserved
%
% For circles
% 10 - radius (m)
%
% For ellipses
% 10 - major radius (m)
% 11 - minor radius (m)
% 12 - orientation of major axis (rad)
%
% For rectangles
% 10 - length (m)
% 11 - height (m)
% 12 - orientation (rad) (relative to x,y already shown)
%
% For lines
% 10 - end point x-axis coordinate relative to start point (m)
% 11 - end point y-axis coordinate relative to start point (m)
%
% For triangles
% 10 - length (m)
% 11 - height (m)
% 12 - offset of peak from midpoint of length (m)
% 13 - orientation (rad)

VCODE=zeros(1,20);		%default - target is not defined

if (state==0)
	return;							%state==0 means that the target is off
end

VCODE(1)=3; %They are rectangles

VCODE(2)=1;							%default is that target is 'on'
VCODE(3)=target_pos(0)*0.01;		%target position in target table is cm (v1.4)
VCODE(4)=target_pos(1)*0.01;		%target position in target table is cm (v1.4)

% Fill colour currently comes from the GUI in 1.x format: RRRGGGBBB. Convert this to a 32-bit 
% 0xRRGGBBAA value, or use zero for transparency if target table index for the colour is zero.
if stateindices(state,1)==0
	VCODE(5)=0;
else
	VCODE(5)=colourshift(target(5));			%fill colour
end

% Stroke colour currently comes from the GUI in 1.x format: RRRGGGBBB. Convert this to a 32-bit 
% 0xRRGGBBAA value, or use zero for transparency if target table index for the colour is zero.
% if stateindices(state,2)==0
% 	VCODE(6)=0;				%if stroke-colour column==0, then stroke colour=0
% else
% 	VCODE(6)=colourshift(target(stateindices(state,2)));			%stroke colour
% end

%if target table index for stroke width is zero, then the stroke width is undefined
% if stateindices(state,3)==0
% 	VCODE(7)=0;					%if stroke-width column==0, then stroke width=0
% elseif stateindices(state,3)<0
% 	VCODE(7)=0.001;			%if stroke is not defined, then a 1mm default is chosen
% else
% 	VCODE(7)=target(stateindices(state,3))*0.01;	%stroke width in target table is cm 
% end

VCODE(10)=target(3)*0.01;       %length (m) -- length in target table is in cm
VCODE(11)=target(4)*0.01;       %height (m) -- height in target table is in cm
% if stateindices(state,6)==0
%     VCODE(12)=0;				%if orientation column==0, then orientation=0
% else
%     VCODE(12)=mod(target(stateindices(state,6)),360)*pi/180.0;  %orientation (rad) -- orientation in target table is degrees (v1.4)
% end

%colourshift converts an RRRGGGBBB colour into an RRGBBAA, as an uint32 
function RRGGBBAA = colourshift(RRRGGGBBB)
	blue = cast(mod(RRRGGGBBB,1000),'uint32');
	green= cast(mod(RRRGGGBBB-blue,1000000)/1000,'uint32');
	red  = cast((RRRGGGBBB-green*1000-blue)/1000000,'uint32');
    RRGGBBAA =   bitshift(red,24)...		% red component
				+ bitshift(green,16)...		% green component
				+ bitshift(blue,8)...		% blue component
				+ 255;						% alpha component

== matlab function Targets1/ShowTarget1 ==
  data: target input inherited; VCODE output inherited; state input inherited
function VCODE  = fcn(target, state)
% This block supports an embeddable subset of the MATLAB language.
% See the help menu for details. 

% VCODEs are length 20.
% All dimensions are units of (m).
% VCODE index definition: 1-5 as the same for all target types
% 1 - Target type
%		1=circle
%		2=ellipse
%       3=rectangle
%		4=line
%       5=triangle
%		6 and higher - not implemented yet
% 2 - status
%		0=off
%		1=on
% 3 - x position (m)
% 4 - y position (m)
% 5 - fill colour
% 6 - stroke colour
% 7 - stroke width
% 8 - reserved
% 9 - reserved
%
% For circles
% 10 - radius (m)
%
% For ellipses
% 10 - major radius (m)
% 11 - minor radius (m)
% 12 - orientation of major axis (rad)
%
% For rectangles
% 10 - length (m)
% 11 - height (m)
% 12 - orientation (rad) (relative to x,y already shown)
%
% For lines
% 10 - end point x-axis coordinate relative to start point (m)
% 11 - end point y-axis coordinate relative to start point (m)
%
% For triangles
% 10 - length (m)
% 11 - height (m)
% 12 - offset of peak from midpoint of length (m)
% 13 - orientation (rad)

VCODE=zeros(1,20);		%default - target is not defined

if (state==0)
	return;							%state==0 means that the target is off
end

VCODE(1)=3; %They are rectangles

VCODE(2)=1;							%default is that target is 'on'
VCODE(3)=target_pos(0)*0.01;		%target position in target table is cm (v1.4)
VCODE(4)=target_pos(1)*0.01;		%target position in target table is cm (v1.4)

% Fill colour currently comes from the GUI in 1.x format: RRRGGGBBB. Convert this to a 32-bit 
% 0xRRGGBBAA value, or use zero for transparency if target table index for the colour is zero.
if stateindices(state,1)==0
	VCODE(5)=0;
else
	VCODE(5)=colourshift(target(5));			%fill colour
end

% Stroke colour currently comes from the GUI in 1.x format: RRRGGGBBB. Convert this to a 32-bit 
% 0xRRGGBBAA value, or use zero for transparency if target table index for the colour is zero.
% if stateindices(state,2)==0
% 	VCODE(6)=0;				%if stroke-colour column==0, then stroke colour=0
% else
% 	VCODE(6)=colourshift(target(stateindices(state,2)));			%stroke colour
% end

%if target table index for stroke width is zero, then the stroke width is undefined
% if stateindices(state,3)==0
% 	VCODE(7)=0;					%if stroke-width column==0, then stroke width=0
% elseif stateindices(state,3)<0
% 	VCODE(7)=0.001;			%if stroke is not defined, then a 1mm default is chosen
% else
% 	VCODE(7)=target(stateindices(state,3))*0.01;	%stroke width in target table is cm 
% end

VCODE(10)=target(3)*0.01;       %length (m) -- length in target table is in cm
VCODE(11)=target(4)*0.01;       %height (m) -- height in target table is in cm
% if stateindices(state,6)==0
%     VCODE(12)=0;				%if orientation column==0, then orientation=0
% else
%     VCODE(12)=mod(target(stateindices(state,6)),360)*pi/180.0;  %orientation (rad) -- orientation in target table is degrees (v1.4)
% end

%colourshift converts an RRRGGGBBB colour into an RRGBBAA, as an uint32 
function RRGGBBAA = colourshift(RRRGGGBBB)
	blue = cast(mod(RRRGGGBBB,1000),'uint32');
	green= cast(mod(RRRGGGBBB-blue,1000000)/1000,'uint32');
	red  = cast((RRRGGGBBB-green*1000-blue)/1000000,'uint32');
    RRGGBBAA =   bitshift(red,24)...		% red component
				+ bitshift(green,16)...		% green component
				+ bitshift(blue,8)...		% blue component
				+ 255;						% alpha component

== matlab function Targets1/ShowTarget2 ==
  data: target input inherited; VCODE output inherited; state input inherited
function VCODE  = fcn(target, state)
% This block supports an embeddable subset of the MATLAB language.
% See the help menu for details. 

% VCODEs are length 20.
% All dimensions are units of (m).
% VCODE index definition: 1-5 as the same for all target types
% 1 - Target type
%		1=circle
%		2=ellipse
%       3=rectangle
%		4=line
%       5=triangle
%		6 and higher - not implemented yet
% 2 - status
%		0=off
%		1=on
% 3 - x position (m)
% 4 - y position (m)
% 5 - fill colour
% 6 - stroke colour
% 7 - stroke width
% 8 - reserved
% 9 - reserved
%
% For circles
% 10 - radius (m)
%
% For ellipses
% 10 - major radius (m)
% 11 - minor radius (m)
% 12 - orientation of major axis (rad)
%
% For rectangles
% 10 - length (m)
% 11 - height (m)
% 12 - orientation (rad) (relative to x,y already shown)
%
% For lines
% 10 - end point x-axis coordinate relative to start point (m)
% 11 - end point y-axis coordinate relative to start point (m)
%
% For triangles
% 10 - length (m)
% 11 - height (m)
% 12 - offset of peak from midpoint of length (m)
% 13 - orientation (rad)

VCODE=zeros(1,20);		%default - target is not defined

if (state==0)
	return;							%state==0 means that the target is off
end

VCODE(1)=3; %They are rectangles

VCODE(2)=1;							%default is that target is 'on'
VCODE(3)=target_pos(0)*0.01;		%target position in target table is cm (v1.4)
VCODE(4)=target_pos(1)*0.01;		%target position in target table is cm (v1.4)

% Fill colour currently comes from the GUI in 1.x format: RRRGGGBBB. Convert this to a 32-bit 
% 0xRRGGBBAA value, or use zero for transparency if target table index for the colour is zero.
if stateindices(state,1)==0
	VCODE(5)=0;
else
	VCODE(5)=colourshift(target(5));			%fill colour
end

% Stroke colour currently comes from the GUI in 1.x format: RRRGGGBBB. Convert this to a 32-bit 
% 0xRRGGBBAA value, or use zero for transparency if target table index for the colour is zero.
% if stateindices(state,2)==0
% 	VCODE(6)=0;				%if stroke-colour column==0, then stroke colour=0
% else
% 	VCODE(6)=colourshift(target(stateindices(state,2)));			%stroke colour
% end

%if target table index for stroke width is zero, then the stroke width is undefined
% if stateindices(state,3)==0
% 	VCODE(7)=0;					%if stroke-width column==0, then stroke width=0
% elseif stateindices(state,3)<0
% 	VCODE(7)=0.001;			%if stroke is not defined, then a 1mm default is chosen
% else
% 	VCODE(7)=target(stateindices(state,3))*0.01;	%stroke width in target table is cm 
% end

VCODE(10)=target(3)*0.01;       %length (m) -- length in target table is in cm
VCODE(11)=target(4)*0.01;       %height (m) -- height in target table is in cm
% if stateindices(state,6)==0
%     VCODE(12)=0;				%if orientation column==0, then orientation=0
% else
%     VCODE(12)=mod(target(stateindices(state,6)),360)*pi/180.0;  %orientation (rad) -- orientation in target table is degrees (v1.4)
% end

%colourshift converts an RRRGGGBBB colour into an RRGBBAA, as an uint32 
function RRGGBBAA = colourshift(RRRGGGBBB)
	blue = cast(mod(RRRGGGBBB,1000),'uint32');
	green= cast(mod(RRRGGGBBB-blue,1000000)/1000,'uint32');
	red  = cast((RRRGGGBBB-green*1000-blue)/1000000,'uint32');
    RRGGBBAA =   bitshift(red,24)...		% red component
				+ bitshift(green,16)...		% green component
				+ bitshift(blue,8)...		% blue component
				+ 255;						% alpha component

== matlab function Targets1/ShowTarget3 ==
  data: target input inherited; VCODE output inherited; state input inherited
function VCODE  = fcn(target, state)
% This block supports an embeddable subset of the MATLAB language.
% See the help menu for details. 

% VCODEs are length 20.
% All dimensions are units of (m).
% VCODE index definition: 1-5 as the same for all target types
% 1 - Target type
%		1=circle
%		2=ellipse
%       3=rectangle
%		4=line
%       5=triangle
%		6 and higher - not implemented yet
% 2 - status
%		0=off
%		1=on
% 3 - x position (m)
% 4 - y position (m)
% 5 - fill colour
% 6 - stroke colour
% 7 - stroke width
% 8 - reserved
% 9 - reserved
%
% For circles
% 10 - radius (m)
%
% For ellipses
% 10 - major radius (m)
% 11 - minor radius (m)
% 12 - orientation of major axis (rad)
%
% For rectangles
% 10 - length (m)
% 11 - height (m)
% 12 - orientation (rad) (relative to x,y already shown)
%
% For lines
% 10 - end point x-axis coordinate relative to start point (m)
% 11 - end point y-axis coordinate relative to start point (m)
%
% For triangles
% 10 - length (m)
% 11 - height (m)
% 12 - offset of peak from midpoint of length (m)
% 13 - orientation (rad)

VCODE=zeros(1,20);		%default - target is not defined

if (state==0)
	return;							%state==0 means that the target is off
end

VCODE(1)=3; %They are rectangles

VCODE(2)=1;							%default is that target is 'on'
VCODE(3)=target_pos(0)*0.01;		%target position in target table is cm (v1.4)
VCODE(4)=target_pos(1)*0.01;		%target position in target table is cm (v1.4)

% Fill colour currently comes from the GUI in 1.x format: RRRGGGBBB. Convert this to a 32-bit 
% 0xRRGGBBAA value, or use zero for transparency if target table index for the colour is zero.
if stateindices(state,1)==0
	VCODE(5)=0;
else
	VCODE(5)=colourshift(target(5));			%fill colour
end

% Stroke colour currently comes from the GUI in 1.x format: RRRGGGBBB. Convert this to a 32-bit 
% 0xRRGGBBAA value, or use zero for transparency if target table index for the colour is zero.
% if stateindices(state,2)==0
% 	VCODE(6)=0;				%if stroke-colour column==0, then stroke colour=0
% else
% 	VCODE(6)=colourshift(target(stateindices(state,2)));			%stroke colour
% end

%if target table index for stroke width is zero, then the stroke width is undefined
% if stateindices(state,3)==0
% 	VCODE(7)=0;					%if stroke-width column==0, then stroke width=0
% elseif stateindices(state,3)<0
% 	VCODE(7)=0.001;			%if stroke is not defined, then a 1mm default is chosen
% else
% 	VCODE(7)=target(stateindices(state,3))*0.01;	%stroke width in target table is cm 
% end

VCODE(10)=target(3)*0.01;       %length (m) -- length in target table is in cm
VCODE(11)=target(4)*0.01;       %height (m) -- height in target table is in cm
% if stateindices(state,6)==0
%     VCODE(12)=0;				%if orientation column==0, then orientation=0
% else
%     VCODE(12)=mod(target(stateindices(state,6)),360)*pi/180.0;  %orientation (rad) -- orientation in target table is degrees (v1.4)
% end

%colourshift converts an RRRGGGBBB colour into an RRGBBAA, as an uint32 
function RRGGBBAA = colourshift(RRRGGGBBB)
	blue = cast(mod(RRRGGGBBB,1000),'uint32');
	green= cast(mod(RRRGGGBBB-blue,1000000)/1000,'uint32');
	red  = cast((RRRGGGBBB-green*1000-blue)/1000000,'uint32');
    RRGGBBAA =   bitshift(red,24)...		% red component
				+ bitshift(green,16)...		% green component
				+ bitshift(blue,8)...		% blue component
				+ 255;						% alpha component
